simulink model "controller_v13"  (R2020b)
settings: Solver=ode4  StartTime=0.0  StopTime=inf  RelTol=1e-3
undefined symbols (not defined in the file): ctr, DiscIntNeverNeededParam, flt, IO397, mdl, rbt, rsim, som, ukf_P0_flat, ukf_prediction_time, ukf_s0, ukf_sys, ukf_use_prediction
libraries: simulink x31, slrealtimeloglib x5, slrealtimeseriallib x5, speedgoatlib_fpga_analog_io x4, slrealtimetgmanagement x3, speedgoatlib_fpga x2, speedgoatlib_fpga_dio x1, slrealtimeutilitieslib x1
(part 2 of 5)

== system controller_v13/Adaptive Controller/ground truth ==
  xyz : Inport
  euler : Inport  Port=2
  f_cmd : Inport  Port=3
  tau_cmd_x : Inport  Port=4
  tau_cmd_y : Inport  Port=5
  gt_state : Inport  Port=6
  Demux : Demux  Outputs=[3, 3, 3, 9, 9, 3, 3, 3]
  Rotm2rpy1 : MATLAB Function  TreatAsAtomicUnit=on
  Terminator{,1..4} (5 alike) : Terminator
  To Workspace2 : ToWorkspace  VariableName=log_est_rpy  SaveFormat=Timeseries  SampleTime=-1
  r : Outport
  r_dot : Outport  Port=2
  r_dotdot : Outport  Port=3
  R : Outport  Port=4
  Omega : Outport  Port=5
  Rdot : Outport  Port=6
  F_ext : Outport  Port=7
  tau_ext : Outport  Port=8
  wires:
  Rotm2rpy1/1(rpy) -> To Workspace2/1
  Demux/4 -> Rotm2rpy1/1(R), R/1
  xyz/1 -> Terminator/1
  euler/1 -> Terminator1/1
  f_cmd/1 -> Terminator2/1
  tau_cmd_x/1 -> Terminator3/1
  tau_cmd_y/1 -> Terminator4/1
  Demux/2 -> r_dot/1
  Demux/3 -> r_dotdot/1
  Demux/7 -> F_ext/1
  Demux/8 -> tau_ext/1
  Demux/6 -> Omega/1
  Demux/5 -> Rdot/1
  Demux/1 -> r/1
  gt_state/1 -> Demux/1

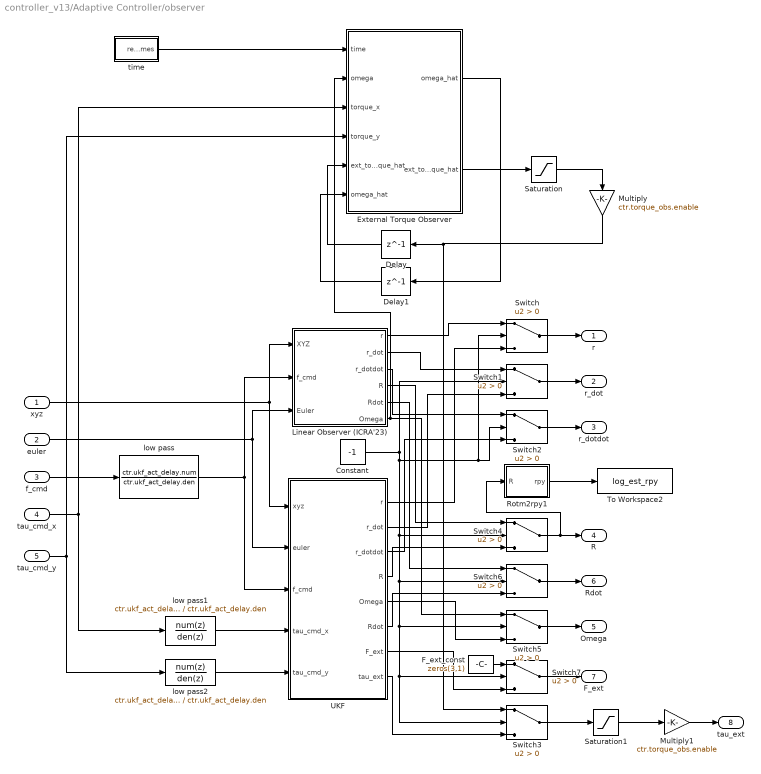
== system controller_v13/Adaptive Controller/observer ==
  xyz : Inport
  euler : Inport  Port=2
  f_cmd : Inport  Port=3
  tau_cmd_x : Inport  Port=4
  tau_cmd_y : Inport  Port=5
  Constant : Constant  Value=-1
  Delay : Delay  DelayLength=1  InitialCondition=[ctr.torque_obs.initial_torque.x; ctr.torque_obs.initial_torque.y; 0.0]  SampleTime=mdl.T
  Delay1 : Delay  DelayLength=1  InitialCondition=[0.0; 0.0]  SampleTime=mdl.T
  External Torque Observer : MATLAB Function  TreatAsAtomicUnit=on
  F_ext_const : Constant  Value=zeros(3,1)
  Linear Observer (ICRA'23) : Subsystem
  Multiply : Gain  Gain=ctr.torque_obs.enable
  Multiply1 : Gain  Gain=ctr.torque_obs.enable
  Rotm2rpy1 : MATLAB Function  TreatAsAtomicUnit=on
  Saturation : Saturate  UpperLimit=1.8*1e-5.*ones(3,1)  LowerLimit=-1.8*1e-5.*ones(3,1)
  Saturation1 : Saturate  UpperLimit=1.8*1e-5.*ones(3,1)  LowerLimit=-1.8*1e-5.*ones(3,1)
  Switch{,1..7} (8 alike) : Switch  Criteria=u2 > Threshold
  To Workspace2 : ToWorkspace  VariableName=log_est_rpy  SaveFormat=Timeseries  SampleTime=-1
  UKF : Subsystem
  low pass : DiscreteTransferFcn  Numerator=ctr.ukf_act_delay.num  Denominator=ctr.ukf_act_delay.den
  low pass1 : DiscreteTransferFcn  Numerator=ctr.ukf_act_delay.num  Denominator=ctr.ukf_act_delay.den
  low pass2 : DiscreteTransferFcn  Numerator=ctr.ukf_act_delay.num  Denominator=ctr.ukf_act_delay.den
  time : Subsystem
  r : Outport
  r_dot : Outport  Port=2
  r_dotdot : Outport  Port=3
  R : Outport  Port=4
  Omega : Outport  Port=5
  Rdot : Outport  Port=6
  F_ext : Outport  Port=7
  tau_ext : Outport  Port=8
  wires:
  UKF/6(Rdot) -> Switch6/3
  UKF/5(Omega) -> Switch5/3
  UKF/3(r_dotdot) -> Switch2/3
  UKF/1(r) -> Switch/3
  UKF/4(R) -> Switch4/3
  UKF/2(r_dot) -> Switch1/3
  Linear Observer (ICRA'23)/6(Omega) -> External Torque Observer/2(omega), Switch5/1
  Linear Observer (ICRA'23)/5(Rdot) -> Switch6/1
  xyz/1 -> Linear Observer (ICRA'23)/1(XYZ), UKF/1(xyz)
  Switch5/1 -> Omega/1
  Linear Observer (ICRA'23)/3(r_dotdot) -> Switch2/1
  Linear Observer (ICRA'23)/4(R) -> Switch4/1
  Linear Observer (ICRA'23)/1(r) -> Switch/1
  Linear Observer (ICRA'23)/2(r_dot) -> Switch1/1
  Switch4/1 -> Rotm2rpy1/1(R), R/1
  Switch2/1 -> r_dotdot/1
  Switch1/1 -> r_dot/1
  Switch/1 -> r/1
  tau_cmd_y/1 -> low pass2/1, External Torque Observer/4(torque_y)
  tau_cmd_x/1 -> External Torque Observer/3(torque_x), low pass1/1
  Constant/1 -> Switch3/2, Switch7/2, Switch5/2, Switch6/2, Switch4/2, Switch2/2, Switch/2, Switch1/2
  euler/1 -> Linear Observer (ICRA'23)/3(Euler), UKF/2(euler)
  f_cmd/1 -> low pass/1
  Rotm2rpy1/1(rpy) -> To Workspace2/1
  Switch6/1 -> Rdot/1
  low pass/1 -> Linear Observer (ICRA'23)/2(f_cmd), UKF/3(f_cmd)
  Switch7/1 -> F_ext/1
  UKF/7(F_ext) -> Switch7/3
  UKF/8(tau_ext) -> Switch3/3
  F_ext_const/1 -> Switch7/1
  External Torque Observer/2(ext_torque_hat) -> Saturation/1
  low pass1/1 -> UKF/4(tau_cmd_x)
  low pass2/1 -> UKF/5(tau_cmd_y)
  Delay1/1 -> External Torque Observer/6("omega_hat ")
  External Torque Observer/1(omega_hat) -> Delay1/1
  time/1(real times) -> External Torque Observer/1(time)
  Delay/1 -> External Torque Observer/5("ext_torque_hat ")
  Saturation/1 -> Multiply/1
  Multiply/1 -> Switch3/1, Delay/1
  Saturation1/1 -> Multiply1/1
  Switch3/1 -> Saturation1/1
  Multiply1/1 -> tau_ext/1

== system controller_v13/Adaptive Controller/time ==
  constant : Constant
  time : DiscreteIntegrator  gainval=1  SampleTime=-1  UpperSaturationLimit=1  LowerSaturationLimit=0  ICPrevOutput=DiscIntNeverNeededParam  ICPrevScaledInput=DiscIntNeverNeededParam
  real times : Outport
  wires:
  constant/1 -> time/1
  time/1 -> real times/1

== system controller_v13/Dynamic Sim/time ==
  constant : Constant
  time : DiscreteIntegrator  gainval=1  SampleTime=-1  UpperSaturationLimit=1  LowerSaturationLimit=0  ICPrevOutput=DiscIntNeverNeededParam  ICPrevScaledInput=DiscIntNeverNeededParam
  real times : Outport
  wires:
  constant/1 -> time/1
  time/1 -> real times/1

== system controller_v13/Force//Torque to Trajectory Specs/force//torque to module thrust ==
  note: No YAW torque control at the moment
  thrust : Inport
  x Tq : Inport  Port=2
  y Tq : Inport  Port=3
  z Tq : Inport  Port=4
  Inputs : slrealtimeloglib/File Log  Commented=on  decimation=1
      settings: SourceProductBaseCode=XP
  Mux : Mux
  SaturatingRamp : DiscreteIntegrator  gainval=1  SampleTime=-1  UpperSaturationLimit=1  LowerSaturationLimit=0  ICPrevOutput=DiscIntNeverNeededParam  ICPrevScaledInput=DiscIntNeverNeededParam
  constant : Constant
  mapping scheme (flipping compataible) : MATLAB Function  TreatAsAtomicUnit=on  SystemSampleTime=mdl.T
  module thrusts (1-4) : Outport  PortDimensions=4
  wires:
  thrust/1 -> Mux/1
  x Tq/1 -> Mux/2
  y Tq/1 -> Mux/3
  z Tq/1 -> Mux/4
  Mux/1 -> Inputs/1, mapping scheme (flipping compataible)/2(inputs)
  mapping scheme (flipping compataible)/1(module_f) -> module thrusts (1-4)/1
  constant/1 -> SaturatingRamp/1
  SaturatingRamp/1 -> mapping scheme (flipping compataible)/1(time)

== system controller_v13/Force//Torque to Trajectory Specs/nominal desired voltage ==
  Force : Inport
  Forces : slrealtimeloglib/File Log  Commented=on  decimation=1
      settings: SourceProductBaseCode=XP
  SaturatingRamp : DiscreteIntegrator  gainval=1  SampleTime=-1  UpperSaturationLimit=1  LowerSaturationLimit=0  ICPrevOutput=DiscIntNeverNeededParam  ICPrevScaledInput=DiscIntNeverNeededParam
  Switch : Switch  Criteria=u2 > Threshold
  constant1 : Constant
  "force to voltage (hovering) " : Subsystem  Commented=on
  force to voltage (sommersault) : Subsystem
  force to voltage flipping : Subsystem
  map_selection : MATLAB Function  TreatAsAtomicUnit=on  SystemSampleTime=mdl.T
  Voltages : Outport
  wires:
  Force/1 -> Forces/1, force to voltage (sommersault)/1(force), force to voltage flipping/1(force)
  force to voltage flipping/1(Vout) -> Switch/3
  Switch/1 -> Voltages/1
  map_selection/1(hover_map) -> Switch/2
  constant1/1 -> SaturatingRamp/1
  SaturatingRamp/1 -> map_selection/1(time)
  force to voltage (sommersault)/1(Vout) -> Switch/1

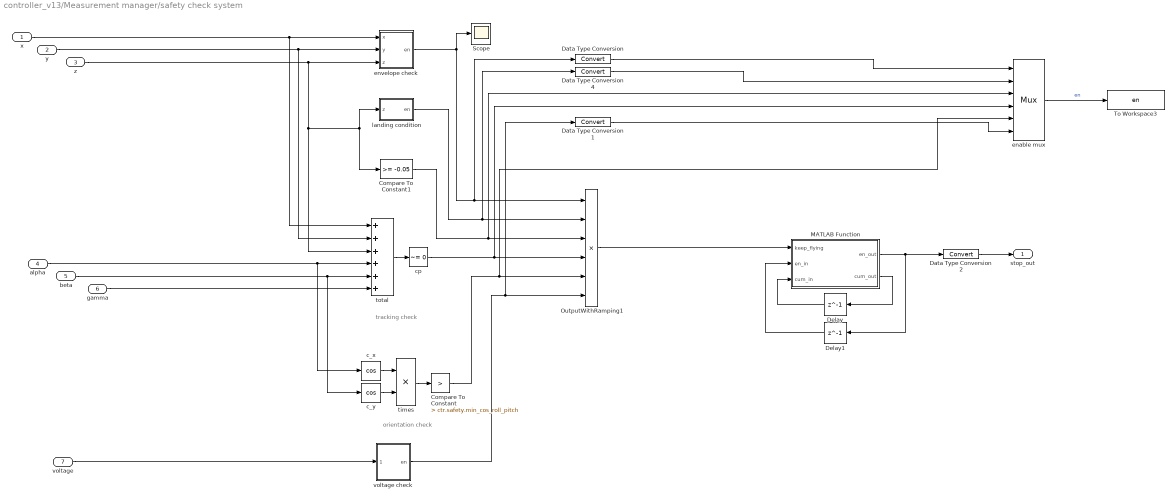
== system controller_v13/Measurement manager/safety check system ==
  note: orientation check
  note: tracking check
  x : Inport
  y : Inport  Port=2
  z : Inport  Port=3
  alpha : Inport  Port=4
  beta : Inport  Port=5
  gamma : Inport  Port=6
  voltage : Inport  Port=7
  Compare To Constant : simulink/Logic and Bit Operations/Compare To Constant  relop=>  const=ctr.safety.min_cos_roll_pitch  OutDataTypeStr=uint8
  Compare To Constant1 : simulink/Logic and Bit Operations/Compare To Constant  relop=>=  const=-0.05  OutDataTypeStr=uint8
  Data Type Conversion{,1..2,4} (4 alike) : DataTypeConversion
  Delay : Delay  DelayLength=1
  Delay1 : Delay  DelayLength=1  InitialCondition=1
  MATLAB Function : MATLAB Function  TreatAsAtomicUnit=on
  OutputWithRamping1 : Product  Inputs=6  RndMeth=Zero
  Scope : Scope
  To Workspace3 : ToWorkspace  VariableName=en  SaveFormat=Timeseries  SampleTime=-1
  c_x : Trigonometry  Operator=cos
  c_y : Trigonometry  Operator=cos
  cp : simulink/Logic and Bit Operations/Compare To Zero  relop=~=  OutDataTypeStr=uint8
  enable mux : Mux  Inputs=6
      settings: DisplayOption=signals
  envelope check : MATLAB Function  TreatAsAtomicUnit=on
  landing condition : Subsystem
  times : Product  RndMeth=Zero
  total : Sum  Inputs=++++++
  voltage check : MATLAB Function  TreatAsAtomicUnit=on  SystemSampleTime=mdl.T
  stop_out : Outport
  wires:
  Compare To Constant1/1 -> enable mux/3, OutputWithRamping1/3
  y/1 -> envelope check/2(y), total/2
  cp/1 -> enable mux/4, OutputWithRamping1/4
  envelope check/1(en) -> Scope/1, Data Type Conversion/1, OutputWithRamping1/1
  enable mux/1 -> To Workspace3/1  "en"
  landing condition/1(en) -> Data Type Conversion4/1, OutputWithRamping1/2
  Data Type Conversion/1 -> enable mux/1
  times/1 -> Compare To Constant/1
  voltage check/1(en) -> Data Type Conversion1/1, OutputWithRamping1/6
  z/1 -> total/3, Compare To Constant1/1, landing condition/1(z), envelope check/3(z)
  Compare To Constant/1 -> enable mux/5, OutputWithRamping1/5
  total/1 -> cp/1
  Data Type Conversion4/1 -> enable mux/2
  x/1 -> total/1, envelope check/1(x)
  alpha/1 -> total/4, c_x/1
  beta/1 -> total/5, c_y/1
  c_x/1 -> times/1
  c_y/1 -> times/2
  Data Type Conversion1/1 -> enable mux/6
  voltage/1 -> voltage check/1(voltage)
  gamma/1 -> total/6
  OutputWithRamping1/1 -> MATLAB Function/1(keep_flying)
  Delay1/1 -> MATLAB Function/2(en_in)
  MATLAB Function/1(en_out) -> Delay1/1, Data Type Conversion2/1
  Delay/1 -> MATLAB Function/3(cum_in)
  MATLAB Function/2(cum_out) -> Delay/1
  Data Type Conversion2/1 -> stop_out/1

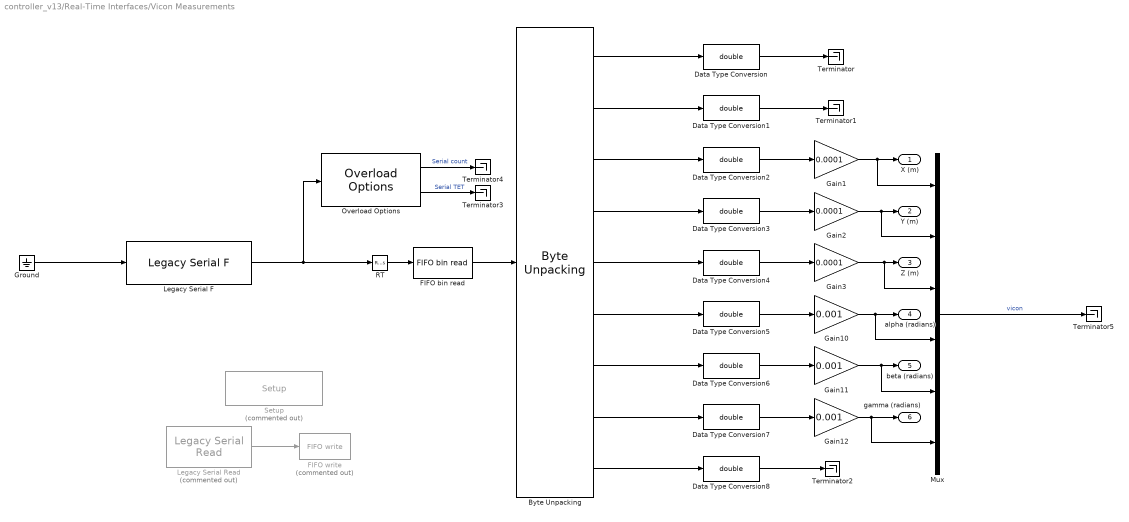
== system controller_v13/Real-Time Interfaces/Vicon Measurements ==
  "Byte Unpacking " : slrealtimeutilitieslib/Byte Unpacking  MaskUnpackedDataTypes={'uint8','int16','int16','int16','int16','int16','int16','int16','uint8'}  MaskUnpackedDataSizes={[1] [1] [1] [1] [1] [1] [1] [1] [1]}  MaskAlignment=1
      settings: SourceProductBaseCode=XP
  Data Type Conversion{,1..8} (9 alike) : DataTypeConversion  OutDataTypeStr=double
  FIFO bin read : slrealtimeseriallib/FIFO bin read  header=[128,127,127]  lengths=[15]  hold=Hold last output if no new data  enable=off  maxsize=15  outputtype=8 bit uint null terminated  sampletime=mdl.T
      settings: SourceProductBaseCode=XP
  FIFO write : slrealtimeseriallib/FIFO write  Commented=on  size=1024  inputtype=count+16 bit uint  present=off  sampletime=-1
      settings: SourceProductBaseCode=XP
  Gain1 : Gain  Gain=0.0001
  Gain10 : Gain  Gain=0.001
  Gain11 : Gain  Gain=0.001
  Gain12 : Gain  Gain=0.001
  Gain2 : Gain  Gain=0.0001
  Gain3 : Gain  Gain=0.0001
  Ground : Ground
  Legacy Serial F : slrealtimeseriallib/Mainboard/Legacy Serial F  port=Legacy Serial Port 1  baud=115200  width=8  nstop=1  parity=None  ctsmode=on  idtype=8 bit uint null terminated  sampletime=0.0005
      settings: SourceProductBaseCode=XP
  Legacy Serial Read : slrealtimeseriallib/Mainboard/Legacy Serial Read  Commented=on  port=Legacy Serial Port 1  count=51  dtype=count+16 bit uint  sampletime=mdl.T
      settings: SourceProductBaseCode=XP
  Mux : Mux  Inputs=6
  Overload Options : slrealtimetgmanagement/Overload Options  startupDur=10  startupDurSrc=Tunable Parameter  maxOverload=10  maxOverloadSrc=Tunable Parameter  TETFlag=on
      settings: SourceProductBaseCode=XP
  RT : RateTransition  Integrity=off  OutPortSampleTime=mdl.T
  Setup : slrealtimeseriallib/Mainboard/Setup  Commented=on  port=Legacy Serial Port 1  baud=115200  width=8  nstop=1  parity=None  ctsmode=on
      settings: SourceProductBaseCode=XP
  Terminator{,1..5} (6 alike) : Terminator
  X (m) : Outport
  Y (m) : Outport  Port=2
  Z (m) : Outport  Port=3
  alpha (radians) : Outport  Port=4
  beta (radians) : Outport  Port=5
  gamma (radians) : Outport  Port=6
  wires:
  "Byte Unpacking "/3 -> Data Type Conversion2/1
  Data Type Conversion2/1 -> Gain1/1
  "Byte Unpacking "/9 -> Data Type Conversion8/1
  "Byte Unpacking "/4 -> Data Type Conversion3/1
  Data Type Conversion6/1 -> Gain11/1
  Data Type Conversion4/1 -> Gain3/1
  "Byte Unpacking "/2 -> Data Type Conversion1/1
  Data Type Conversion5/1 -> Gain10/1
  Data Type Conversion7/1 -> Gain12/1
  "Byte Unpacking "/6 -> Data Type Conversion5/1
  "Byte Unpacking "/8 -> Data Type Conversion7/1
  Data Type Conversion3/1 -> Gain2/1
  "Byte Unpacking "/5 -> Data Type Conversion4/1
  "Byte Unpacking "/7 -> Data Type Conversion6/1
  "Byte Unpacking "/1 -> Data Type Conversion/1
  Gain1/1 -> Mux/1, X (m)/1
  Gain2/1 -> Mux/2, Y (m)/1
  Gain3/1 -> Mux/3, Z (m)/1
  Gain10/1 -> Mux/4, alpha (radians)/1
  Gain11/1 -> Mux/5, beta (radians)/1
  Gain12/1 -> Mux/6, gamma (radians)/1
  Legacy Serial Read/1 -> FIFO write/1
  FIFO bin read/1 -> "Byte Unpacking "/1
  Ground/1 -> Legacy Serial F/1
  Legacy Serial F/1 -> Overload Options/1, RT/1
  RT/1 -> FIFO bin read/1
  Data Type Conversion/1 -> Terminator/1
  Data Type Conversion1/1 -> Terminator1/1
  Data Type Conversion8/1 -> Terminator2/1
  Mux/1 -> Terminator5/1  "vicon"
  Overload Options/1 -> Terminator4/1  "Serial count"
  Overload Options/2 -> Terminator3/1  "Serial TET"

== system controller_v13/Real-Time Interfaces/z Amplifier Measurement ==
  IO397 Analog Input : speedgoatlib_fpga_analog_io/IO397 Analog Input  Commented=on  id=1  chan=[1:4]  range=+-10.24 V  trigger=Initiator  ts=mdl.T_high  pciSlot=[6,0]  board=IO397-50k
      settings: SourceProductName=Simulink Real-Time: Speedgoat Library
  IO397 Analog Input1 : speedgoatlib_fpga_analog_io/IO397 Analog Input  Commented=on  id=2  chan=[1:4]  range=+-10.24 V  trigger=Initiator  ts=mdl.T_high  pciSlot=[11,0]  board=IO397-50k
      settings: SourceProductName=Simulink Real-Time: Speedgoat Library
  Mux : Mux  Commented=on  Inputs=8
  Overload Options : slrealtimetgmanagement/Overload Options  Commented=on  startupDur=10  startupDurSrc=Tunable Parameter  maxOverload=1000  maxOverloadSrc=Tunable Parameter  TETFlag=on
      settings: SourceProductBaseCode=XP
  Terminator1 : Terminator  Commented=on
  Terminator2 : Terminator  Commented=on
  wires:
  IO397 Analog Input/4 -> Mux/4
  IO397 Analog Input/2 -> Mux/2
  IO397 Analog Input/1 -> Mux/1
  IO397 Analog Input/3 -> Mux/3
  IO397 Analog Input1/1 -> Mux/5
  IO397 Analog Input1/2 -> Mux/6
  IO397 Analog Input1/3 -> Mux/7
  IO397 Analog Input1/4 -> Mux/8
  Mux/1 -> Overload Options/1
  Overload Options/1 -> Terminator2/1  "Sensing count"
  Overload Options/2 -> Terminator1/1  "Sensing TET"

== system controller_v13/closed loop en/safety1 ==
  In1 : Inport
  Compare To Constant1 : simulink/Logic and Bit Operations/Compare To Constant  relop=<=  const=inf  OutDataTypeStr=uint8
  Switch1 : Switch  Threshold=0.5
  zero1 : Constant  Value=0
  Out1 : Outport
  wires:
  In1/1 -> Switch1/1, Compare To Constant1/1
  Compare To Constant1/1 -> Switch1/2
  zero1/1 -> Switch1/3
  Switch1/1 -> Out1/1

== system controller_v13/closed loop en/safety2 ==
  In1 : Inport
  Compare To Constant1 : simulink/Logic and Bit Operations/Compare To Constant  relop=<=  const=inf  OutDataTypeStr=uint8
  Switch1 : Switch  Threshold=0.5
  zero1 : Constant  Value=0
  Out1 : Outport
  wires:
  In1/1 -> Switch1/1, Compare To Constant1/1
  Compare To Constant1/1 -> Switch1/2
  zero1/1 -> Switch1/3
  Switch1/1 -> Out1/1

== system controller_v13/closed loop en/safety3 ==
  In1 : Inport
  Compare To Constant1 : simulink/Logic and Bit Operations/Compare To Constant  relop=<=  const=inf  OutDataTypeStr=uint8
  Switch1 : Switch  Threshold=0.5
  zero1 : Constant  Value=0
  Out1 : Outport
  wires:
  In1/1 -> Switch1/1, Compare To Constant1/1
  Compare To Constant1/1 -> Switch1/2
  zero1/1 -> Switch1/3
  Switch1/1 -> Out1/1

== system controller_v13/closed loop en/safety4 ==
  In1 : Inport
  Compare To Constant1 : simulink/Logic and Bit Operations/Compare To Constant  relop=<=  const=inf  OutDataTypeStr=uint8
  Switch1 : Switch  Threshold=0.5
  zero1 : Constant  Value=0
  Out1 : Outport
  wires:
  In1/1 -> Switch1/1, Compare To Constant1/1
  Compare To Constant1/1 -> Switch1/2
  zero1/1 -> Switch1/3
  Switch1/1 -> Out1/1

== system controller_v13/signal generator/Bias_Signal ==
  note: time constant = 0.002sec
  QuasiEnable : Inport
  BiasVolts : Inport  Port=2
  AveragedBias : Subsystem
  PreGain : Gain
  Product : Product  RndMeth=Zero
  SIgnalForRamp_binary : Subsystem
  SaturatingRamp : DiscreteIntegrator  gainval=10  SampleTime=-1  LimitOutput=on  UpperSaturationLimit=1  LowerSaturationLimit=0  ICPrevOutput=DiscIntNeverNeededParam  ICPrevScaledInput=DiscIntNeverNeededParam
  BiasD2A : Outport
  wires:
  PreGain/1 -> BiasD2A/1
  BiasVolts/1 -> AveragedBias/1(In1)
  QuasiEnable/1 -> SIgnalForRamp_binary/1(In1)
  SIgnalForRamp_binary/1(Out1) -> SaturatingRamp/1
  SaturatingRamp/1 -> Product/1
  AveragedBias/1(Out1) -> Product/2
  Product/1 -> PreGain/1

== system controller_v13/signal generator/Drive_Signal1 ==
  QuasiEnable : Inport
  Frequency : Inport  Port=2
  Offset : Inport  Port=3
  Amplitude : Inport  Port=4
  PitchBias : Inport  Port=5
  split cycle mu : Inport  Port=6
  AveragedAmp_filtered : Subsystem
  AveragedOffset_filtered : Subsystem
  AveragedTau_filtered : Subsystem
  OutputWithRamping : Product  RndMeth=Zero
  PreGain : Constant
  PrescaledAmp : Product  RndMeth=Zero
  PrescaledOffset : Product  RndMeth=Zero
  ProductPhase : Product  RndMeth=Zero
  RampUpOrDown : DiscreteIntegrator  gainval=10  SampleTime=-1  LimitOutput=on  UpperSaturationLimit=1  LowerSaturationLimit=0  ICPrevOutput=DiscIntNeverNeededParam  ICPrevScaledInput=DiscIntNeverNeededParam
  SignalForRamp_binary : Subsystem
  SignalForSin_binary : Subsystem
  Subsystem : Subsystem
  Sum : Sum
  Sum1 : Sum
  signal with gain : Product  RndMeth=Zero
  SignalOutput : Outport
  WithoutRamp : Outport  Port=2
  RampOutput : Outport  Port=3
  AmplitudeOutput : Outport  Port=4
  OffsetOutput : Outport  Port=5
  wires:
  PrescaledAmp/1 -> AveragedAmp_filtered/1(In1)
  Sum/1 -> OutputWithRamping/2, WithoutRamp/1
  RampUpOrDown/1 -> RampOutput/1, OutputWithRamping/1, SignalForSin_binary/1(In1)
  QuasiEnable/1 -> SignalForRamp_binary/1(In1)
  SignalForRamp_binary/1(Out1) -> RampUpOrDown/1
  Amplitude/1 -> PrescaledAmp/1
  signal with gain/1 -> Sum/1
  Frequency/1 -> ProductPhase/2
  SignalForSin_binary/1(Out1) -> ProductPhase/1
  ProductPhase/1 -> Subsystem/2(In2)
  AveragedOffset_filtered/1(Out1) -> Sum/2, OffsetOutput/1
  PrescaledOffset/1 -> AveragedOffset_filtered/1(In1)
  PreGain/1 -> PrescaledAmp/2, PrescaledOffset/2
  OutputWithRamping/1 -> SignalOutput/1
  AveragedAmp_filtered/1(Out1) -> signal with gain/2, AmplitudeOutput/1
  Sum1/1 -> PrescaledOffset/1
  Offset/1 -> Sum1/1
  PitchBias/1 -> Sum1/2
  AveragedTau_filtered/1(Out1) -> Subsystem/1(split cycle mu)
  split cycle mu/1 -> AveragedTau_filtered/1(In1)
  Subsystem/1(split cycle signal) -> signal with gain/1

== system controller_v13/signal generator/Drive_Signal2 ==
  QuasiEnable : Inport
  Frequency : Inport  Port=2
  Offset : Inport  Port=3
  Amplitude : Inport  Port=4
  PitchBias : Inport  Port=5
  split cycle mu : Inport  Port=6
  AveragedAmp_filtered : Subsystem
  AveragedOffset_filtered : Subsystem
  AveragedTau_filtered : Subsystem
  OutputWithRamping : Product  RndMeth=Zero
  PreGain : Constant
  PrescaledAmp : Product  RndMeth=Zero
  PrescaledOffset : Product  RndMeth=Zero
  ProductPhase : Product  RndMeth=Zero
  RampUpOrDown : DiscreteIntegrator  gainval=10  SampleTime=-1  LimitOutput=on  UpperSaturationLimit=1  LowerSaturationLimit=0  ICPrevOutput=DiscIntNeverNeededParam  ICPrevScaledInput=DiscIntNeverNeededParam
  SignalForRamp_binary : Subsystem
  SignalForSin_binary : Subsystem
  Subsystem : Subsystem
  Sum : Sum
  Sum1 : Sum
  signal with gain : Product  RndMeth=Zero
  SignalOutput : Outport
  WithoutRamp : Outport  Port=2
  RampOutput : Outport  Port=3
  AmplitudeOutput : Outport  Port=4
  OffsetOutput : Outport  Port=5
  wires:
  PrescaledAmp/1 -> AveragedAmp_filtered/1(In1)
  Sum/1 -> OutputWithRamping/2, WithoutRamp/1
  RampUpOrDown/1 -> RampOutput/1, OutputWithRamping/1, SignalForSin_binary/1(In1)
  QuasiEnable/1 -> SignalForRamp_binary/1(In1)
  SignalForRamp_binary/1(Out1) -> RampUpOrDown/1
  Amplitude/1 -> PrescaledAmp/1
  signal with gain/1 -> Sum/1
  Frequency/1 -> ProductPhase/2
  SignalForSin_binary/1(Out1) -> ProductPhase/1
  ProductPhase/1 -> Subsystem/2(In2)
  AveragedOffset_filtered/1(Out1) -> Sum/2, OffsetOutput/1
  PrescaledOffset/1 -> AveragedOffset_filtered/1(In1)
  PreGain/1 -> PrescaledAmp/2, PrescaledOffset/2
  OutputWithRamping/1 -> SignalOutput/1
  AveragedAmp_filtered/1(Out1) -> signal with gain/2, AmplitudeOutput/1
  Sum1/1 -> PrescaledOffset/1
  Offset/1 -> Sum1/1
  PitchBias/1 -> Sum1/2
  AveragedTau_filtered/1(Out1) -> Subsystem/1(split cycle mu)
  split cycle mu/1 -> AveragedTau_filtered/1(In1)
  Subsystem/1(split cycle signal) -> signal with gain/1

== system controller_v13/signal generator/Drive_Signal3 ==
  QuasiEnable : Inport
  Frequency : Inport  Port=2
  Offset : Inport  Port=3
  Amplitude : Inport  Port=4
  PitchBias : Inport  Port=5
  split cycle mu : Inport  Port=6
  AveragedAmp_filtered : Subsystem
  AveragedOffset_filtered : Subsystem
  AveragedTau_filtered : Subsystem
  OutputWithRamping : Product  RndMeth=Zero
  PreGain : Constant
  PrescaledAmp : Product  RndMeth=Zero
  PrescaledOffset : Product  RndMeth=Zero
  ProductPhase : Product  RndMeth=Zero
  RampUpOrDown : DiscreteIntegrator  gainval=10  SampleTime=-1  LimitOutput=on  UpperSaturationLimit=1  LowerSaturationLimit=0  ICPrevOutput=DiscIntNeverNeededParam  ICPrevScaledInput=DiscIntNeverNeededParam
  SignalForRamp_binary : Subsystem
  SignalForSin_binary : Subsystem
  Subsystem : Subsystem
  Sum : Sum
  Sum1 : Sum
  signal with gain : Product  RndMeth=Zero
  SignalOutput : Outport
  WithoutRamp : Outport  Port=2
  RampOutput : Outport  Port=3
  AmplitudeOutput : Outport  Port=4
  OffsetOutput : Outport  Port=5
  wires:
  PrescaledAmp/1 -> AveragedAmp_filtered/1(In1)
  Sum/1 -> OutputWithRamping/2, WithoutRamp/1
  RampUpOrDown/1 -> RampOutput/1, OutputWithRamping/1, SignalForSin_binary/1(In1)
  QuasiEnable/1 -> SignalForRamp_binary/1(In1)
  SignalForRamp_binary/1(Out1) -> RampUpOrDown/1
  Amplitude/1 -> PrescaledAmp/1
  signal with gain/1 -> Sum/1
  Frequency/1 -> ProductPhase/2
  SignalForSin_binary/1(Out1) -> ProductPhase/1
  ProductPhase/1 -> Subsystem/2(In2)
  AveragedOffset_filtered/1(Out1) -> Sum/2, OffsetOutput/1
  PrescaledOffset/1 -> AveragedOffset_filtered/1(In1)
  PreGain/1 -> PrescaledAmp/2, PrescaledOffset/2
  OutputWithRamping/1 -> SignalOutput/1
  AveragedAmp_filtered/1(Out1) -> signal with gain/2, AmplitudeOutput/1
  Sum1/1 -> PrescaledOffset/1
  Offset/1 -> Sum1/1
  PitchBias/1 -> Sum1/2
  AveragedTau_filtered/1(Out1) -> Subsystem/1(split cycle mu)
  split cycle mu/1 -> AveragedTau_filtered/1(In1)
  Subsystem/1(split cycle signal) -> signal with gain/1

== system controller_v13/signal generator/Drive_Signal4 ==
  QuasiEnable : Inport
  Frequency : Inport  Port=2
  Offset : Inport  Port=3
  Amplitude : Inport  Port=4
  PitchBias : Inport  Port=5
  split cycle mu : Inport  Port=6
  AveragedAmp_filtered : Subsystem
  AveragedOffset_filtered : Subsystem
  AveragedTau_filtered : Subsystem
  OutputWithRamping : Product  RndMeth=Zero
  PreGain : Constant
  PrescaledAmp : Product  RndMeth=Zero
  PrescaledOffset : Product  RndMeth=Zero
  ProductPhase : Product  RndMeth=Zero
  RampUpOrDown : DiscreteIntegrator  gainval=10  SampleTime=-1  LimitOutput=on  UpperSaturationLimit=1  LowerSaturationLimit=0  ICPrevOutput=DiscIntNeverNeededParam  ICPrevScaledInput=DiscIntNeverNeededParam
  SignalForRamp_binary : Subsystem
  SignalForSin_binary : Subsystem
  Subsystem : Subsystem
  Sum : Sum
  Sum1 : Sum
  signal with gain : Product  RndMeth=Zero
  SignalOutput : Outport
  WithoutRamp : Outport  Port=2
  RampOutput : Outport  Port=3
  AmplitudeOutput : Outport  Port=4
  OffsetOutput : Outport  Port=5
  wires:
  PrescaledAmp/1 -> AveragedAmp_filtered/1(In1)
  Sum/1 -> OutputWithRamping/2, WithoutRamp/1
  RampUpOrDown/1 -> RampOutput/1, OutputWithRamping/1, SignalForSin_binary/1(In1)
  QuasiEnable/1 -> SignalForRamp_binary/1(In1)
  SignalForRamp_binary/1(Out1) -> RampUpOrDown/1
  Amplitude/1 -> PrescaledAmp/1
  signal with gain/1 -> Sum/1
  Frequency/1 -> ProductPhase/2
  SignalForSin_binary/1(Out1) -> ProductPhase/1
  ProductPhase/1 -> Subsystem/2(In2)
  AveragedOffset_filtered/1(Out1) -> Sum/2, OffsetOutput/1
  PrescaledOffset/1 -> AveragedOffset_filtered/1(In1)
  PreGain/1 -> PrescaledAmp/2, PrescaledOffset/2
  OutputWithRamping/1 -> SignalOutput/1
  AveragedAmp_filtered/1(Out1) -> signal with gain/2, AmplitudeOutput/1
  Sum1/1 -> PrescaledOffset/1
  Offset/1 -> Sum1/1
  PitchBias/1 -> Sum1/2
  AveragedTau_filtered/1(Out1) -> Subsystem/1(split cycle mu)
  split cycle mu/1 -> AveragedTau_filtered/1(In1)
  Subsystem/1(split cycle signal) -> signal with gain/1

== system controller_v13/signal generator/SignalSaturationLimit ==
  BiasMax : Inport
  SignalRaw : Inport  Port=2
  GainBias : Gain
  MaxOf : MinMax  Function=max  Inputs=2
  MinOf : MinMax  Inputs=2
  ground : Constant
  SignalSatd : Outport
  wires:
  BiasMax/1 -> GainBias/1
  SignalRaw/1 -> MinOf/2
  MinOf/1 -> MaxOf/1
  MaxOf/1 -> SignalSatd/1
  GainBias/1 -> MinOf/1
  ground/1 -> MaxOf/2

== system controller_v13/signal generator/SignalSaturationLimit1 ==
  BiasMax : Inport
  SignalRaw : Inport  Port=2
  GainBias : Gain
  MaxOf : MinMax  Function=max  Inputs=2
  MinOf : MinMax  Inputs=2
  ground : Constant
  SignalSatd : Outport
  wires:
  BiasMax/1 -> GainBias/1
  SignalRaw/1 -> MinOf/2
  MinOf/1 -> MaxOf/1
  MaxOf/1 -> SignalSatd/1
  GainBias/1 -> MinOf/1
  ground/1 -> MaxOf/2

== system controller_v13/signal generator/SignalSaturationLimit2 ==
  BiasMax : Inport
  SignalRaw : Inport  Port=2
  GainBias : Gain
  MaxOf : MinMax  Function=max  Inputs=2
  MinOf : MinMax  Inputs=2
  ground : Constant
  SignalSatd : Outport
  wires:
  BiasMax/1 -> GainBias/1
  SignalRaw/1 -> MinOf/2
  MinOf/1 -> MaxOf/1
  MaxOf/1 -> SignalSatd/1
  GainBias/1 -> MinOf/1
  ground/1 -> MaxOf/2

== system controller_v13/signal generator/SignalSaturationLimit3 ==
  BiasMax : Inport
  SignalRaw : Inport  Port=2
  GainBias : Gain
  MaxOf : MinMax  Function=max  Inputs=2
  MinOf : MinMax  Inputs=2
  ground : Constant
  SignalSatd : Outport
  wires:
  BiasMax/1 -> GainBias/1
  SignalRaw/1 -> MinOf/2
  MinOf/1 -> MaxOf/1
  MaxOf/1 -> SignalSatd/1
  GainBias/1 -> MinOf/1
  ground/1 -> MaxOf/2

== system controller_v13/Adaptive Controller/Attitude and thrust learned NMPC/time ==
  constant : Constant
  time : DiscreteIntegrator  gainval=1  SampleTime=-1  UpperSaturationLimit=1  LowerSaturationLimit=0  ICPrevOutput=DiscIntNeverNeededParam  ICPrevScaledInput=DiscIntNeverNeededParam
  real times : Outport
  wires:
  constant/1 -> time/1
  time/1 -> real times/1

== system controller_v13/Adaptive Controller/ICRA'23 attitude and thrust MPC controller -> It works/time ==
  constant : Constant
  time : DiscreteIntegrator  gainval=1  SampleTime=-1  UpperSaturationLimit=1  LowerSaturationLimit=0  ICPrevOutput=DiscIntNeverNeededParam  ICPrevScaledInput=DiscIntNeverNeededParam
  real times : Outport
  wires:
  constant/1 -> time/1
  time/1 -> real times/1

== system controller_v13/Adaptive Controller/adaptive system/integrator ==
  note: integrator limit (saturation) needs to be set.
  e : Inport
  torque offset : Inport  Port=2
  thrust_offset : Inport  Port=3
  enable1 : Product  Inputs=**
  initial guess : MATLAB Function  TreatAsAtomicUnit=on
  integrator with sat : DiscreteIntegrator  IntegratorMethod=Integration: Backward Euler  gainval=1  SampleTime=-1  LimitOutput=on  UpperSaturationLimit=ctr.integral.lim.upper  LowerSaturationLimit=ctr.integral.lim.lower  ICPrevOutput=DiscIntNeverNeededParam  ICPrevScaledInput=DiscIntNeverNeededParam
  safety2 : Subsystem
  start ramp : Subsystem
  int_e : Outport
  " torq_off" : Outport  Port=2
  th_off : Outport  Port=3
  wires:
  safety2/1(Out1) -> enable1/2
  enable1/1 -> integrator with sat/1
  start ramp/1(Out1) -> enable1/1
  e/1 -> safety2/1(In1)
  integrator with sat/1 -> initial guess/1(i_e)
  initial guess/1(int_e) -> int_e/1
  initial guess/2(tor_inte) -> " torq_off"/1
  initial guess/3(th_inte) -> th_off/1
  torque offset/1 -> initial guess/2(tor_off)
  thrust_offset/1 -> initial guess/3(th_off)

== system controller_v13/Adaptive Controller/adaptive system/safety1 ==
  In1 : Inport
  Compare To Constant1 : simulink/Logic and Bit Operations/Compare To Constant  relop=<=  const=inf  OutDataTypeStr=uint8
  Switch1 : Switch  Threshold=0.5
  zero1 : Constant  Value=0
  Out1 : Outport
  wires:
  In1/1 -> Switch1/1, Compare To Constant1/1
  Compare To Constant1/1 -> Switch1/2
  zero1/1 -> Switch1/3
  Switch1/1 -> Out1/1

== system controller_v13/Adaptive Controller/adaptive system/safety2 ==
  In1 : Inport
  Compare To Constant1 : simulink/Logic and Bit Operations/Compare To Constant  relop=<=  const=inf  OutDataTypeStr=uint8
  Switch1 : Switch  Threshold=0.5
  zero1 : Constant  Value=0
  Out1 : Outport
  wires:
  In1/1 -> Switch1/1, Compare To Constant1/1
  Compare To Constant1/1 -> Switch1/2
  zero1/1 -> Switch1/3
  Switch1/1 -> Out1/1

== system controller_v13/Adaptive Controller/attitude and thrust MPC controller2/NN RTMPC ==
  time : Inport
  r : Inport  Port=2
  r_dot : Inport  Port=3
  r_dotdot : Inport  Port=4
  R : Inport  Port=5
  Omega : Inport  Port=6
  rd : Inport  Port=7
  rd_d : Inport  Port=8
  rd_dd : Inport  Port=9
  rd_ddd : Inport  Port=10
  rd_dddd : Inport  Port=11
  int_e : Inport  Port=12
  MATLAB Function : MATLAB Function  TreatAsAtomicUnit=on
  MATLAB Function1 : MATLAB Function  TreatAsAtomicUnit=on
  MATLAB Function2 : MATLAB Function  TreatAsAtomicUnit=on
  Normalize NN Inputs : Gain  Gain=1/10
  Normalize NN Outputs : Gain  Gain=12
  Rd : Outport
  Omegad : Outport  Port=2
  cmd_B_acc_z : Outport  Port=3
  alt_e : Outport  Port=4
  wires:
  MATLAB Function1/1(Rd) -> Rd/1
  rd/1 -> MATLAB Function/7(rd)
  MATLAB Function1/4(alt_e) -> alt_e/1
  MATLAB Function1/2(Omegad) -> Omegad/1
  rd_d/1 -> MATLAB Function/8(rd_d)
  rd_dddd/1 -> MATLAB Function/11(rd_dddd)
  MATLAB Function1/3(cmd_B_acc_z) -> cmd_B_acc_z/1
  r_dotdot/1 -> MATLAB Function/4(r_dotdot)
  r_dot/1 -> MATLAB Function/3(r_dot)
  MATLAB Function/1(x_in) -> Normalize NN Inputs/1
  int_e/1 -> MATLAB Function/12(int_e)
  time/1 -> MATLAB Function/1(time)
  rd_dd/1 -> MATLAB Function/9(rd_dd)
  rd_ddd/1 -> MATLAB Function/10(rd_ddd)
  Omega/1 -> MATLAB Function/6(Omega)
  r/1 -> MATLAB Function/2(r)
  R/1 -> MATLAB Function1/2(R), MATLAB Function/5(R)
  Normalize NN Inputs/1 -> MATLAB Function2/1(x)
  Normalize NN Outputs/1 -> MATLAB Function1/1(u_nn)
  MATLAB Function2/1(y) -> Normalize NN Outputs/1

== system controller_v13/Adaptive Controller/attitude and thrust MPC controller2/time ==
  constant : Constant
  time : DiscreteIntegrator  gainval=1  SampleTime=-1  UpperSaturationLimit=1  LowerSaturationLimit=0  ICPrevOutput=DiscIntNeverNeededParam  ICPrevScaledInput=DiscIntNeverNeededParam
  real times : Outport
  wires:
  constant/1 -> time/1
  time/1 -> real times/1

== system controller_v13/Adaptive Controller/observer/Linear Observer (ICRA'23) ==
  XYZ : Inport
  f_cmd : Inport  Port=2
  Euler : Inport  Port=3
  Rotaion : Subsystem
  Terminator : Terminator
  Terminator1 : Terminator
  Terminator2 : Terminator
  lateral KF observer : Subsystem
  lateral observer : Subsystem  Commented=on
  r : Outport
  r_dot : Outport  Port=2
  r_dotdot : Outport  Port=3
  R : Outport  Port=4
  Rdot : Outport  Port=5
  Omega : Outport  Port=6
  wires:
  Rotaion/2(Rdot) -> Rdot/1
  lateral observer/1(r) -> Terminator/1
  Rotaion/1(R) -> R/1, lateral KF observer/1(R)
  Rotaion/3(Omega) -> Omega/1
  lateral observer/2(r_dot) -> Terminator1/1
  XYZ/1 -> lateral KF observer/3(xyz), lateral observer/1(XYZ)
  lateral KF observer/1(r) -> r/1
  lateral KF observer/2(r_dot) -> r_dot/1
  f_cmd/1 -> lateral KF observer/2(f_cmd)
  lateral observer/3(r_dotdot) -> Terminator2/1
  Euler/1 -> Rotaion/1(Euler)
  lateral KF observer/3(r_dotdot) -> r_dotdot/1

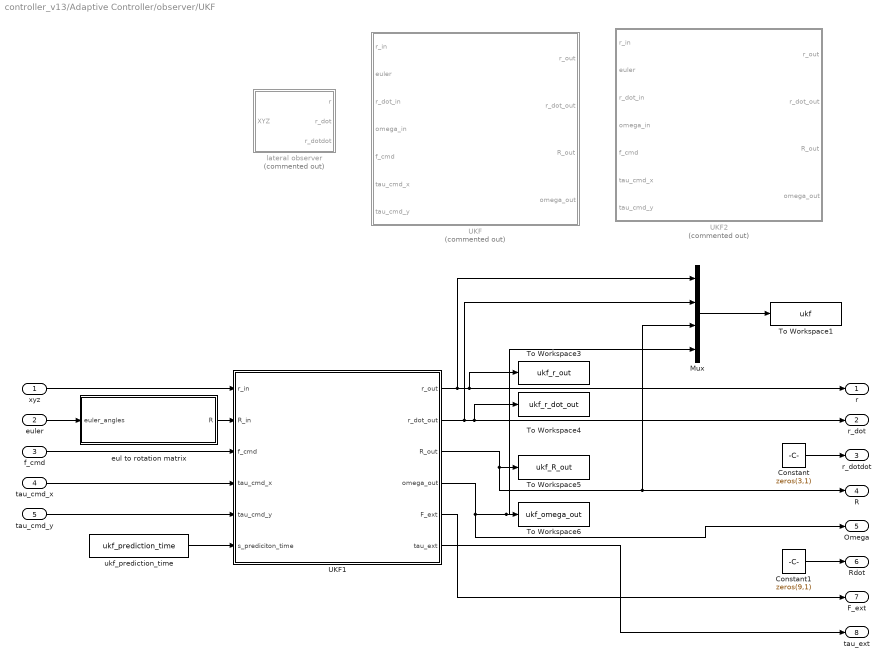
== system controller_v13/Adaptive Controller/observer/UKF ==
  xyz : Inport
  euler : Inport  Port=2
  f_cmd : Inport  Port=3
  tau_cmd_x : Inport  Port=4
  tau_cmd_y : Inport  Port=5
  Constant : Constant  Value=zeros(3,1)
  Constant1 : Constant  Value=zeros(9,1)
  Mux : Mux
  To Workspace1 : ToWorkspace  VariableName=ukf  SaveFormat=Timeseries  SampleTime=-1
  To Workspace3 : ToWorkspace  VariableName=ukf_r_out  SaveFormat=Timeseries  SampleTime=-1
  To Workspace4 : ToWorkspace  VariableName=ukf_r_dot_out  SaveFormat=Timeseries  SampleTime=-1
  To Workspace5 : ToWorkspace  VariableName=ukf_R_out  SaveFormat=Timeseries  SampleTime=-1
  To Workspace6 : ToWorkspace  VariableName=ukf_omega_out  SaveFormat=Timeseries  SampleTime=-1
  UKF : Subsystem  Commented=on
  UKF1 : Subsystem
  UKF2 : Subsystem  Commented=on
  eul to rotation matrix : MATLAB Function  TreatAsAtomicUnit=on
  lateral observer : Subsystem  Commented=on
  ukf_prediction_time : Constant  Value=ukf_prediction_time
  r : Outport
  r_dot : Outport  Port=2
  r_dotdot : Outport  Port=3
  R : Outport  Port=4
  Omega : Outport  Port=5
  Rdot : Outport  Port=6
  F_ext : Outport  Port=7
  tau_ext : Outport  Port=8
  wires:
  euler/1 -> eul to rotation matrix/1(euler_angles)
  xyz/1 -> UKF1/1(r_in)
  UKF1/4(omega_out) -> Omega/1, Mux/4, To Workspace6/1
  UKF1/3(R_out) -> Mux/3, R/1, To Workspace5/1
  UKF1/2(r_dot_out) -> To Workspace4/1, r_dot/1, Mux/2
  UKF1/1(r_out) -> To Workspace3/1, r/1, Mux/1
  Constant1/1 -> Rdot/1
  Mux/1 -> To Workspace1/1
  ukf_prediction_time/1 -> UKF1/6(s_prediciton_time)
  Constant/1 -> r_dotdot/1
  eul to rotation matrix/1(R) -> UKF1/2(R_in)
  f_cmd/1 -> UKF1/3(f_cmd)
  tau_cmd_x/1 -> UKF1/4(tau_cmd_x)
  tau_cmd_y/1 -> UKF1/5(tau_cmd_y)
  UKF1/5(F_ext) -> F_ext/1
  UKF1/6(tau_ext) -> tau_ext/1

== system controller_v13/Adaptive Controller/observer/time ==
  constant : Constant
  time : DiscreteIntegrator  gainval=1  SampleTime=-1  UpperSaturationLimit=1  LowerSaturationLimit=0  ICPrevOutput=DiscIntNeverNeededParam  ICPrevScaledInput=DiscIntNeverNeededParam
  real times : Outport
  wires:
  constant/1 -> time/1
  time/1 -> real times/1

== system controller_v13/Force//Torque to Trajectory Specs/nominal desired voltage/force to voltage (hovering)  ==
  note: apply max voltage limit
  note: known correction from open-loop tests
  force : Inport
  Add : Sum  Inputs=+++
  Constant : Constant  Value=rbt.VM_input1
  Constant1 : Constant  Value=rbt.DV
  Constant2 : Constant  Value=rbt.VM_input2
  MATLAB Function : MATLAB Function  TreatAsAtomicUnit=on
  Product : Product
  Vout : Outport
  wires:
  MATLAB Function/1(Vo) -> Vout/1
  force/1 -> Product/2
  Constant2/1 -> Add/2
  Product/1 -> Add/3
  Add/1 -> MATLAB Function/1(Vi)
  Constant1/1 -> Add/1
  Constant/1 -> Product/1

== system controller_v13/Force//Torque to Trajectory Specs/nominal desired voltage/force to voltage (sommersault) ==
  note: apply max voltage limit
  note: known correction from open-loop tests
  force : Inport
  Add : Sum
  Constant1 : Constant  Value=rbt.DV
  MATLAB Function : MATLAB Function  TreatAsAtomicUnit=on
  MATLAB Function1 : MATLAB Function  TreatAsAtomicUnit=on
  Vout : Outport
  wires:
  MATLAB Function/1(Vo) -> Vout/1
  MATLAB Function1/1(y) -> Add/2
  Add/1 -> MATLAB Function/1(Vi)
  Constant1/1 -> Add/1
  force/1 -> MATLAB Function1/1(u)

== system controller_v13/Force//Torque to Trajectory Specs/nominal desired voltage/force to voltage flipping ==
  note: apply max voltage limit
  note: known correction from open-loop tests
  force : Inport
  Add : Sum
  Constant : Constant  Value=rbt.VM2
  Constant1 : Constant  Value=rbt.DV_flip
  MATLAB Function : MATLAB Function  TreatAsAtomicUnit=on
  Product : Product
  Sqrt : Sqrt  SaturateOnIntegerOverflow=on
  Vout : Outport
  wires:
  MATLAB Function/1(Vo) -> Vout/1
  force/1 -> Sqrt/1
  Add/1 -> MATLAB Function/1(Vi)
  Constant1/1 -> Add/1
  Constant/1 -> Product/1
  Product/1 -> Add/2
  Sqrt/1 -> Product/2

== system controller_v13/Measurement manager/safety check system/landing condition ==
  z : Inport
  Add : Sum  Inputs=+--
  SaturatingRamp1 : DiscreteIntegrator  gainval=1  SampleTime=-1  UpperSaturationLimit=1  LowerSaturationLimit=0  ICPrevOutput=DiscIntNeverNeededParam  ICPrevScaledInput=DiscIntNeverNeededParam
  constant : Constant
  constant1 : Constant  Value=2
  constant2 : Constant  Value=mdl.i_delay
  landing_cond : MATLAB Function  TreatAsAtomicUnit=on  SystemSampleTime=mdl.T
  en : Outport
  wires:
  SaturatingRamp1/1 -> Add/1
  constant/1 -> SaturatingRamp1/1
  constant1/1 -> Add/2
  constant2/1 -> Add/3
  Add/1 -> landing_cond/2(time_cond)
  z/1 -> landing_cond/1(alt)
  landing_cond/1(en) -> en/1

== system controller_v13/signal generator/Bias_Signal/AveragedBias ==
  note: To avoid having signal "jump",
      | we want SMOOTH transitions
      | in frequency (i.e., a weighted sum
      | of current freq and freq some delta t ago)
  note: time constant = 0.002sec
  In1 : Inport
  Discrete Transfer Fcn : DiscreteTransferFcn  Numerator=[0.05]  Denominator=[1 -.95]
  Out1 : Outport
  wires:
  In1/1 -> Discrete Transfer Fcn/1
  Discrete Transfer Fcn/1 -> Out1/1

== system controller_v13/signal generator/Bias_Signal/SIgnalForRamp_binary ==
  note: Should output 1 or -1,
      | so signal ramps UP to 1
      | or DOWN to 0.
  In1 : Inport
  Add : Sum  Inputs=+-
  Compare To Zero : simulink/Logic and Bit Operations/Compare To Zero  relop=>  OutDataTypeStr=uint8  ZeroCross=off
  Constant : Constant
  Data Type Conversion : DataTypeConversion  OutDataTypeStr=double
  Gain : Gain  Gain=2
  Out1 : Outport
  wires:
  In1/1 -> Compare To Zero/1
  Compare To Zero/1 -> Data Type Conversion/1
  Gain/1 -> Add/1
  Constant/1 -> Add/2
  Add/1 -> Out1/1
  Data Type Conversion/1 -> Gain/1

== system controller_v13/signal generator/Drive_Signal1/AveragedAmp_filtered ==
  note: To avoid having signal "jump",
      | we want SMOOTH transitions
      | in frequency (i.e., a weighted sum
      | of current freq and freq some delta t ago)
  note: time constant 0.002sec
      | for 10kHz samping
  In1 : Inport
  Discrete Transfer Fcn : DiscreteTransferFcn  Numerator=[0.05]  Denominator=[1 -.95]
  Out1 : Outport
  wires:
  In1/1 -> Discrete Transfer Fcn/1
  Discrete Transfer Fcn/1 -> Out1/1

== system controller_v13/signal generator/Drive_Signal1/AveragedOffset_filtered ==
  note: To avoid having signal "jump",
      | we want SMOOTH transitions
      | in frequency (i.e., a weighted sum
      | of current freq and freq some delta t ago)
  note: c
  note: time constant 0.02sec
      | for 10kHz samping
  In1 : Inport
  Discrete Transfer Fcn : DiscreteTransferFcn  Numerator=[0.05]  Denominator=[1 -.95]
  Out1 : Outport
  wires:
  In1/1 -> Discrete Transfer Fcn/1
  Discrete Transfer Fcn/1 -> Out1/1

== system controller_v13/signal generator/Drive_Signal1/AveragedTau_filtered ==
  note: To avoid having signal "jump",
      | we want SMOOTH transitions
      | in frequency (i.e., a weighted sum
      | of current freq and freq some delta t ago)
  note: time constant 0.002sec
      | for 10kHz samping
  In1 : Inport
  Discrete Transfer Fcn : DiscreteTransferFcn  Numerator=[0.05]  Denominator=[1, -0.95]
  Out1 : Outport
  wires:
  In1/1 -> Discrete Transfer Fcn/1
  Discrete Transfer Fcn/1 -> Out1/1

== system controller_v13/signal generator/Drive_Signal1/SignalForRamp_binary ==
  note: Should output 1 or -1,
      | so signal ramps UP to 1
      | or DOWN to 0.
  In1 : Inport
  Add : Sum  Inputs=+-
  Compare To Zero : simulink/Logic and Bit Operations/Compare To Zero  relop=>  OutDataTypeStr=uint8  ZeroCross=off
  Constant : Constant
  Data Type Conversion : DataTypeConversion  OutDataTypeStr=double
  Gain : Gain  Gain=2
  Out1 : Outport
  wires:
  In1/1 -> Compare To Zero/1
  Compare To Zero/1 -> Data Type Conversion/1
  Gain/1 -> Add/1
  Constant/1 -> Add/2
  Add/1 -> Out1/1
  Data Type Conversion/1 -> Gain/1

== system controller_v13/signal generator/Drive_Signal1/SignalForSin_binary ==
  note: We want this to stay "high" for 1
      | second after the actual "enable"
      | is turned off...
  In1 : Inport
  Compare To Zero : simulink/Logic and Bit Operations/Compare To Zero  relop=>  OutDataTypeStr=uint8  ZeroCross=off
  Data Type Conversion : DataTypeConversion  OutDataTypeStr=double
  Out1 : Outport
  wires:
  In1/1 -> Compare To Zero/1
  Compare To Zero/1 -> Data Type Conversion/1
  Data Type Conversion/1 -> Out1/1

== system controller_v13/signal generator/Drive_Signal1/Subsystem ==
  note: positive value pushes the left wing forward
  split cycle mu : Inport
  In2 : Inport  Port=2
  1-mu : Sum  Inputs=+-
  2f : Gain  Gain=2
  2nd harmonic : Trigonometry  OutputSignalType=real
  2pi : Gain  Gain=2*pi
  Abs1 : Abs
  Add : Sum
  Constant : Constant
  combined sines : Sum
  deg to rad : Gain  Gain=pi/180
  f : Gain  Gain=-1
  first harmonic : Trigonometry  OutputSignalType=real
  omega*t : DiscreteIntegrator  SampleTime=-1  ICPrevOutput=DiscIntNeverNeededParam  ICPrevScaledInput=DiscIntNeverNeededParam
  phase offset : Constant  Value=0
  signal with gain1 : Product  RndMeth=Zero
  signal with gain2 : Product  RndMeth=Zero
  split cycle signal : Outport
  wires:
  2f/1 -> 2nd harmonic/1
  first harmonic/1 -> signal with gain1/2
  Constant/1 -> 1-mu/1
  split cycle mu/1 -> f/1, Abs1/1
  1-mu/1 -> signal with gain1/1
  2nd harmonic/1 -> signal with gain2/2
  signal with gain1/1 -> combined sines/1
  signal with gain2/1 -> combined sines/2
  combined sines/1 -> split cycle signal/1
  f/1 -> signal with gain2/1
  Abs1/1 -> 1-mu/2
  In2/1 -> 2pi/1
  2pi/1 -> omega*t/1
  omega*t/1 -> Add/2
  Add/1 -> first harmonic/1, 2f/1
  phase offset/1 -> deg to rad/1
  deg to rad/1 -> Add/1

== system controller_v13/signal generator/Drive_Signal2/AveragedAmp_filtered ==
  note: To avoid having signal "jump",
      | we want SMOOTH transitions
      | in frequency (i.e., a weighted sum
      | of current freq and freq some delta t ago)
  note: time constant 0.002sec
      | for 10kHz samping
  In1 : Inport
  Discrete Transfer Fcn : DiscreteTransferFcn  Numerator=[0.05]  Denominator=[1 -.95]
  Out1 : Outport
  wires:
  In1/1 -> Discrete Transfer Fcn/1
  Discrete Transfer Fcn/1 -> Out1/1

== system controller_v13/signal generator/Drive_Signal2/AveragedOffset_filtered ==
  note: To avoid having signal "jump",
      | we want SMOOTH transitions
      | in frequency (i.e., a weighted sum
      | of current freq and freq some delta t ago)
  note: c
  note: time constant 0.02sec
      | for 10kHz samping
  In1 : Inport
  Discrete Transfer Fcn : DiscreteTransferFcn  Numerator=[0.05]  Denominator=[1 -.95]
  Out1 : Outport
  wires:
  In1/1 -> Discrete Transfer Fcn/1
  Discrete Transfer Fcn/1 -> Out1/1

== system controller_v13/signal generator/Drive_Signal2/AveragedTau_filtered ==
  note: To avoid having signal "jump",
      | we want SMOOTH transitions
      | in frequency (i.e., a weighted sum
      | of current freq and freq some delta t ago)
  note: time constant 0.002sec
      | for 10kHz samping
  In1 : Inport
  Discrete Transfer Fcn : DiscreteTransferFcn  Numerator=[0.05]  Denominator=[1, -0.95]
  Out1 : Outport
  wires:
  In1/1 -> Discrete Transfer Fcn/1
  Discrete Transfer Fcn/1 -> Out1/1

== system controller_v13/signal generator/Drive_Signal2/SignalForRamp_binary ==
  note: Should output 1 or -1,
      | so signal ramps UP to 1
      | or DOWN to 0.
  In1 : Inport
  Add : Sum  Inputs=+-
  Compare To Zero : simulink/Logic and Bit Operations/Compare To Zero  relop=>  OutDataTypeStr=uint8  ZeroCross=off
  Constant : Constant
  Data Type Conversion : DataTypeConversion  OutDataTypeStr=double
  Gain : Gain  Gain=2
  Out1 : Outport
  wires:
  In1/1 -> Compare To Zero/1
  Compare To Zero/1 -> Data Type Conversion/1
  Gain/1 -> Add/1
  Constant/1 -> Add/2
  Add/1 -> Out1/1
  Data Type Conversion/1 -> Gain/1

== system controller_v13/signal generator/Drive_Signal2/SignalForSin_binary ==
  note: We want this to stay "high" for 1
      | second after the actual "enable"
      | is turned off...
  In1 : Inport
  Compare To Zero : simulink/Logic and Bit Operations/Compare To Zero  relop=>  OutDataTypeStr=uint8  ZeroCross=off
  Data Type Conversion : DataTypeConversion  OutDataTypeStr=double
  Out1 : Outport
  wires:
  In1/1 -> Compare To Zero/1
  Compare To Zero/1 -> Data Type Conversion/1
  Data Type Conversion/1 -> Out1/1

== system controller_v13/signal generator/Drive_Signal2/Subsystem ==
  note: positive value pushes the left wing forward
  split cycle mu : Inport
  In2 : Inport  Port=2
  1-mu : Sum  Inputs=+-
  2f : Gain  Gain=2
  2nd harmonic : Trigonometry  OutputSignalType=real
  2pi : Gain  Gain=2*pi
  Abs1 : Abs
  Add : Sum
  Constant : Constant
  combined sines : Sum
  deg to rad : Gain  Gain=pi/180
  f : Gain  Gain=-1
  first harmonic : Trigonometry  OutputSignalType=real
  omega*t : DiscreteIntegrator  SampleTime=-1  ICPrevOutput=DiscIntNeverNeededParam  ICPrevScaledInput=DiscIntNeverNeededParam
  phase offset : Constant  Value=180
  signal with gain1 : Product  RndMeth=Zero
  signal with gain2 : Product  RndMeth=Zero
  split cycle signal : Outport
  wires:
  2f/1 -> 2nd harmonic/1
  first harmonic/1 -> signal with gain1/2
  Constant/1 -> 1-mu/1
  split cycle mu/1 -> f/1, Abs1/1
  1-mu/1 -> signal with gain1/1
  2nd harmonic/1 -> signal with gain2/2
  signal with gain1/1 -> combined sines/1
  signal with gain2/1 -> combined sines/2
  combined sines/1 -> split cycle signal/1
  f/1 -> signal with gain2/1
  Abs1/1 -> 1-mu/2
  In2/1 -> 2pi/1
  2pi/1 -> omega*t/1
  omega*t/1 -> Add/2
  Add/1 -> first harmonic/1, 2f/1
  phase offset/1 -> deg to rad/1
  deg to rad/1 -> Add/1

== system controller_v13/signal generator/Drive_Signal3/AveragedAmp_filtered ==
  note: To avoid having signal "jump",
      | we want SMOOTH transitions
      | in frequency (i.e., a weighted sum
      | of current freq and freq some delta t ago)
  note: time constant 0.002sec
      | for 10kHz samping
  In1 : Inport
  Discrete Transfer Fcn : DiscreteTransferFcn  Numerator=[0.05]  Denominator=[1 -.95]
  Out1 : Outport
  wires:
  In1/1 -> Discrete Transfer Fcn/1
  Discrete Transfer Fcn/1 -> Out1/1

== system controller_v13/signal generator/Drive_Signal3/AveragedOffset_filtered ==
  note: To avoid having signal "jump",
      | we want SMOOTH transitions
      | in frequency (i.e., a weighted sum
      | of current freq and freq some delta t ago)
  note: c
  note: time constant 0.02sec
      | for 10kHz samping
  In1 : Inport
  Discrete Transfer Fcn : DiscreteTransferFcn  Numerator=[0.05]  Denominator=[1 -.95]
  Out1 : Outport
  wires:
  In1/1 -> Discrete Transfer Fcn/1
  Discrete Transfer Fcn/1 -> Out1/1

== system controller_v13/signal generator/Drive_Signal3/AveragedTau_filtered ==
  note: To avoid having signal "jump",
      | we want SMOOTH transitions
      | in frequency (i.e., a weighted sum
      | of current freq and freq some delta t ago)
  note: time constant 0.002sec
      | for 10kHz samping
  In1 : Inport
  Discrete Transfer Fcn : DiscreteTransferFcn  Numerator=[0.05]  Denominator=[1 -.95]
  Out1 : Outport
  wires:
  In1/1 -> Discrete Transfer Fcn/1
  Discrete Transfer Fcn/1 -> Out1/1

== system controller_v13/signal generator/Drive_Signal3/SignalForRamp_binary ==
  note: Should output 1 or -1,
      | so signal ramps UP to 1
      | or DOWN to 0.
  In1 : Inport
  Add : Sum  Inputs=+-
  Compare To Zero : simulink/Logic and Bit Operations/Compare To Zero  relop=>  OutDataTypeStr=uint8  ZeroCross=off
  Constant : Constant
  Data Type Conversion : DataTypeConversion  OutDataTypeStr=double
  Gain : Gain  Gain=2
  Out1 : Outport
  wires:
  In1/1 -> Compare To Zero/1
  Compare To Zero/1 -> Data Type Conversion/1
  Gain/1 -> Add/1
  Constant/1 -> Add/2
  Add/1 -> Out1/1
  Data Type Conversion/1 -> Gain/1

== system controller_v13/signal generator/Drive_Signal3/SignalForSin_binary ==
  note: We want this to stay "high" for 1
      | second after the actual "enable"
      | is turned off...
  In1 : Inport
  Compare To Zero : simulink/Logic and Bit Operations/Compare To Zero  relop=>  OutDataTypeStr=uint8  ZeroCross=off
  Data Type Conversion : DataTypeConversion  OutDataTypeStr=double
  Out1 : Outport
  wires:
  In1/1 -> Compare To Zero/1
  Compare To Zero/1 -> Data Type Conversion/1
  Data Type Conversion/1 -> Out1/1

== system controller_v13/signal generator/Drive_Signal3/Subsystem ==
  split cycle mu : Inport
  In2 : Inport  Port=2
  1-mu : Sum  Inputs=+-
  2f : Gain  Gain=2
  2nd harmonic : Trigonometry  OutputSignalType=real
  2pi : Gain  Gain=2*pi
  Abs1 : Abs
  Constant : Constant
  SmoothClock : DiscreteIntegrator  SampleTime=-1  ICPrevOutput=DiscIntNeverNeededParam  ICPrevScaledInput=DiscIntNeverNeededParam
  combined sines : Sum
  f : Gain
  first harmonic : Trigonometry  OutputSignalType=real
  signal with gain1 : Product  RndMeth=Zero
  signal with gain2 : Product  RndMeth=Zero
  split cycle signal : Outport
  wires:
  SmoothClock/1 -> first harmonic/1, 2f/1
  2f/1 -> 2nd harmonic/1
  2pi/1 -> SmoothClock/1
  first harmonic/1 -> signal with gain1/2
  Constant/1 -> 1-mu/1
  split cycle mu/1 -> f/1, Abs1/1
  1-mu/1 -> signal with gain1/1
  2nd harmonic/1 -> signal with gain2/2
  signal with gain1/1 -> combined sines/1
  signal with gain2/1 -> combined sines/2
  combined sines/1 -> split cycle signal/1
  In2/1 -> 2pi/1
  f/1 -> signal with gain2/1
  Abs1/1 -> 1-mu/2
